simulink model "c00002"  (R2018a)
settings: Solver=FixedStepAuto  StartTime=0.0  StopTime=300  FixedStep=0.1  RelTol=1e-3
undefined symbols (not defined in the file): A1, hmax, R1, R2, TempThreshold
settings Model: Creator=aarrieta  LastModifiedBy=umarkiegi

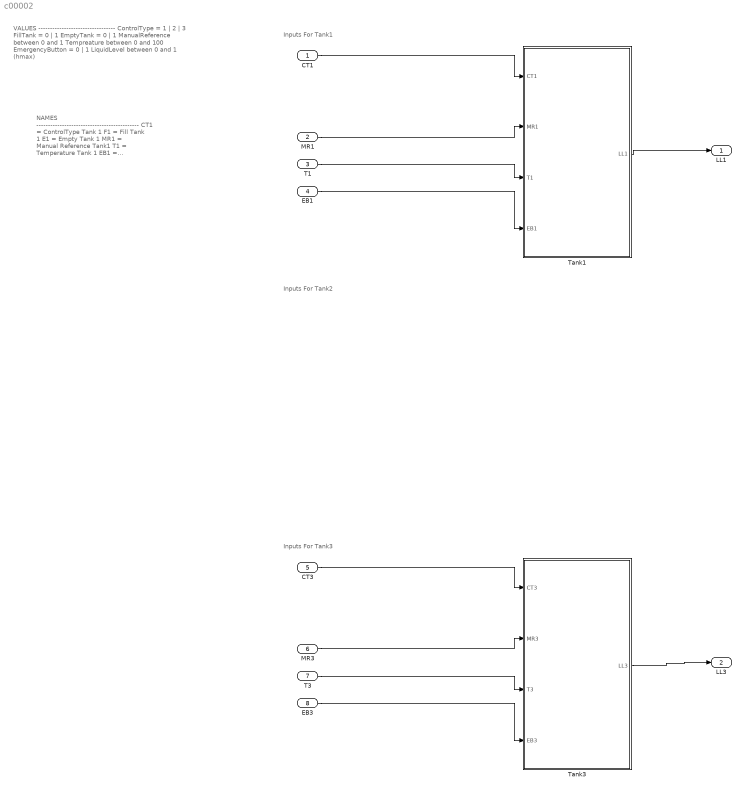
== system c00002 ==
  note: Inputs For Tank1
  note: VALUES
      | ---------------------------------
      | ControlType = 1 | 2 | 3
      | FillTank = 0 | 1
      | EmptyTank = 0 | 1
      | ManualReference between 0 and 1
      | Tempreature between 0 and 100
      | EmergencyButton = 0 | 1
      | LiquidLevel between 0 and 1 (hmax)
  note: NAMES
      | --------------------------------------------
      | CT1 = ControlType Tank 1
      | F1 = Fill Tank 1
      | E1 = Empty Tank 1
      | MR1 = Manual Reference Tank1
      | T1 = Temperature Tank 1
      | EB1 = Emergency Button Tank 1
      | LL1 = Liquid Level 1
  note: Inputs For Tank2
  note: Inputs For Tank3
  CT1 : Inport
  MR1 : Inport  Port=2
  T1 : Inport  Port=3
  EB1 : Inport  Port=4
  CT3 : Inport  Port=5
  MR3 : Inport  Port=6
  T3 : Inport  Port=7
  EB3 : Inport  Port=8
  Tank1 : Subsystem
  Tank3 : Subsystem
  LL1 : Outport
  LL3 : Outport  Port=2
  wires:
  Tank1/1(LL1) -> LL1/1
  CT1/1 -> Tank1/1(CT1)
  MR1/1 -> Tank1/2(MR1)
  T1/1 -> Tank1/3(T1)
  EB1/1 -> Tank1/4(EB1)
  Tank3/1(LL3) -> LL3/1
  MR3/1 -> Tank3/2(MR3)
  T3/1 -> Tank3/3(T3)
  EB3/1 -> Tank3/4(EB3)
  CT3/1 -> Tank3/1(CT3)

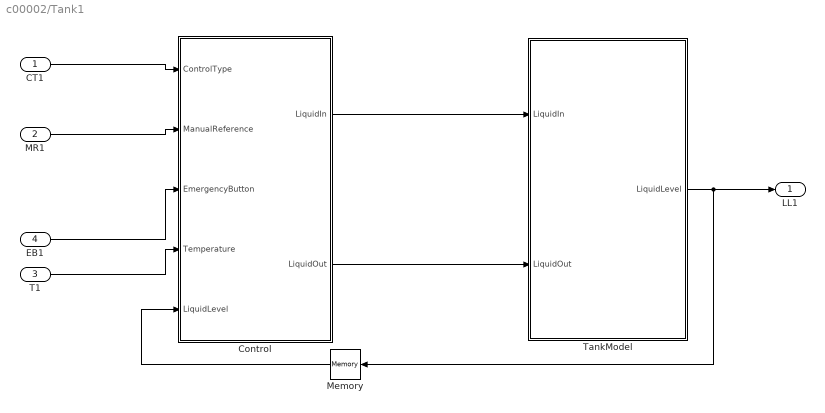
== system c00002/Tank1 ==
  CT1 : Inport
  MR1 : Inport  Port=2
  T1 : Inport  Port=3
  EB1 : Inport  Port=4
  Control : Subsystem
  Memory : Memory
  TankModel : Subsystem
  LL1 : Outport
  wires:
  TankModel/1(LiquidLevel) -> Memory/1, LL1/1
  Control/2(LiquidOut) -> TankModel/2(LiquidOut)
  Memory/1 -> Control/5(LiquidLevel)
  MR1/1 -> Control/2(ManualReference)
  CT1/1 -> Control/1(ControlType)
  EB1/1 -> Control/3(EmergencyButton)
  T1/1 -> Control/4(Temperature)
  Control/1(LiquidIn) -> TankModel/1(LiquidIn)

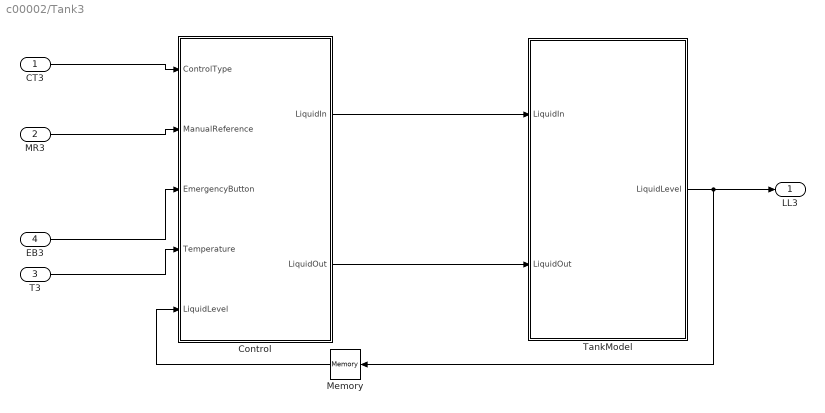
== system c00002/Tank3 ==
  CT3 : Inport
  MR3 : Inport  Port=2
  T3 : Inport  Port=3
  EB3 : Inport  Port=4
  Control : Subsystem
  Memory : Memory
  TankModel : Subsystem
  LL3 : Outport
  wires:
  TankModel/1(LiquidLevel) -> Memory/1, LL3/1
  Control/2(LiquidOut) -> TankModel/2(LiquidOut)
  Memory/1 -> Control/5(LiquidLevel)
  MR3/1 -> Control/2(ManualReference)
  CT3/1 -> Control/1(ControlType)
  EB3/1 -> Control/3(EmergencyButton)
  T3/1 -> Control/4(Temperature)
  Control/1(LiquidIn) -> TankModel/1(LiquidIn)

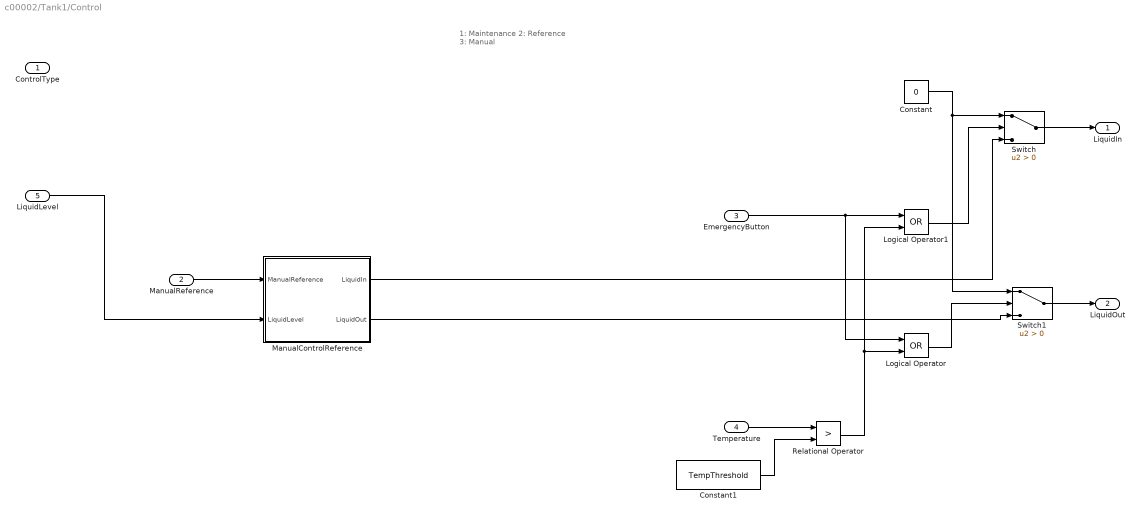
== system c00002/Tank1/Control ==
  note: 1: Maintenance
      | 2: Reference
      | 3: Manual
  ControlType : Inport
  ManualReference : Inport  Port=2
  EmergencyButton : Inport  Port=3
  Temperature : Inport  Port=4
  LiquidLevel : Inport  Port=5
  Constant : Constant  Value=0
  Constant1 : Constant  Value=TempThreshold
  Logical Operator : Logic  Operator=OR  AllPortsSameDT=off  OutDataTypeStr=boolean
  Logical Operator1 : Logic  Operator=OR  AllPortsSameDT=off  OutDataTypeStr=boolean
  ManualControlReference : Subsystem
  Relational Operator : RelationalOperator  Operator=>  OutDataTypeStr=boolean  RndMeth=Simplest
  Switch : Switch  Criteria=u2 > Threshold
  Switch1 : Switch  Criteria=u2 > Threshold
  LiquidIn : Outport
  LiquidOut : Outport  Port=2
  wires:
  ManualReference/1 -> ManualControlReference/1(ManualReference)
  LiquidLevel/1 -> ManualControlReference/2(LiquidLevel)
  Switch/1 -> LiquidIn/1
  Switch1/1 -> LiquidOut/1
  Constant/1 -> Switch1/1, Switch/1
  EmergencyButton/1 -> Logical Operator/1, Logical Operator1/1
  Relational Operator/1 -> Logical Operator1/2, Logical Operator/2
  Logical Operator/1 -> Switch1/2
  Logical Operator1/1 -> Switch/2
  Temperature/1 -> Relational Operator/1
  Constant1/1 -> Relational Operator/2
  ManualControlReference/1(LiquidIn) -> Switch/3
  ManualControlReference/2(LiquidOut) -> Switch1/3

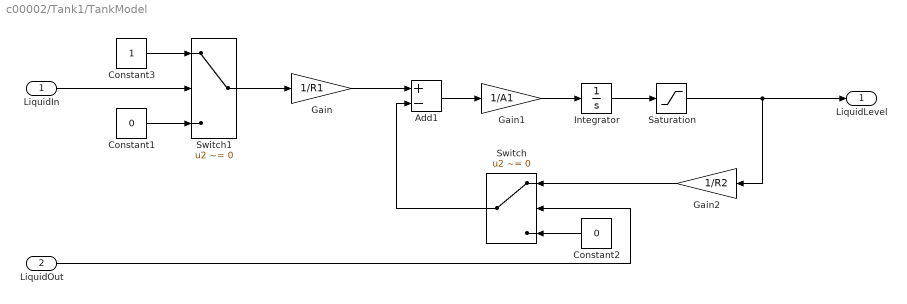
== system c00002/Tank1/TankModel ==
  LiquidIn : Inport
  LiquidOut : Inport  Port=2
  Add1 : Sum  Inputs=+-
  Constant1 : Constant  Value=0
  Constant2 : Constant  Value=0
  Constant3 : Constant
  Gain : Gain  Gain=1/R1
  Gain1 : Gain  Gain=1/A1
  Gain2 : Gain  Gain=1/R2
  Integrator : Integrator
  Saturation : Saturate  UpperLimit=hmax  LowerLimit=0
  Switch : Switch  Criteria=u2 ~= 0
  Switch1 : Switch  Criteria=u2 ~= 0
  LiquidLevel : Outport
  wires:
  Saturation/1 -> LiquidLevel/1, Gain2/1
  LiquidOut/1 -> Switch/2
  Add1/1 -> Gain1/1
  Gain2/1 -> Switch/1
  LiquidIn/1 -> Switch1/2
  Switch/1 -> Add1/2
  Switch1/1 -> Gain/1
  Constant2/1 -> Switch/3
  Constant3/1 -> Switch1/1
  Integrator/1 -> Saturation/1
  Gain1/1 -> Integrator/1
  Gain/1 -> Add1/1
  Constant1/1 -> Switch1/3

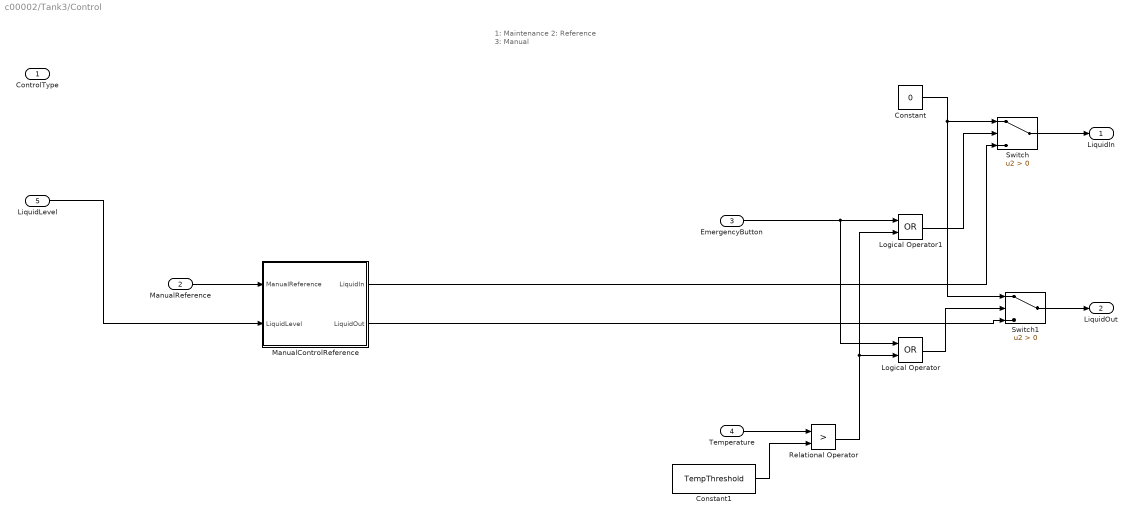
== system c00002/Tank3/Control ==
  note: 1: Maintenance
      | 2: Reference
      | 3: Manual
  ControlType : Inport
  ManualReference : Inport  Port=2
  EmergencyButton : Inport  Port=3
  Temperature : Inport  Port=4
  LiquidLevel : Inport  Port=5
  Constant : Constant  Value=0
  Constant1 : Constant  Value=TempThreshold
  Logical Operator : Logic  Operator=OR  AllPortsSameDT=off  OutDataTypeStr=boolean
  Logical Operator1 : Logic  Operator=OR  AllPortsSameDT=off  OutDataTypeStr=boolean
  ManualControlReference : Subsystem
  Relational Operator : RelationalOperator  Operator=>  OutDataTypeStr=boolean  RndMeth=Simplest
  Switch : Switch  Criteria=u2 > Threshold
  Switch1 : Switch  Criteria=u2 > Threshold
  LiquidIn : Outport
  LiquidOut : Outport  Port=2
  wires:
  ManualReference/1 -> ManualControlReference/1(ManualReference)
  LiquidLevel/1 -> ManualControlReference/2(LiquidLevel)
  Switch/1 -> LiquidIn/1
  Switch1/1 -> LiquidOut/1
  Constant/1 -> Switch1/1, Switch/1
  EmergencyButton/1 -> Logical Operator/1, Logical Operator1/1
  Relational Operator/1 -> Logical Operator1/2, Logical Operator/2
  Logical Operator/1 -> Switch1/2
  Logical Operator1/1 -> Switch/2
  Temperature/1 -> Relational Operator/1
  Constant1/1 -> Relational Operator/2
  ManualControlReference/1(LiquidIn) -> Switch/3
  ManualControlReference/2(LiquidOut) -> Switch1/3

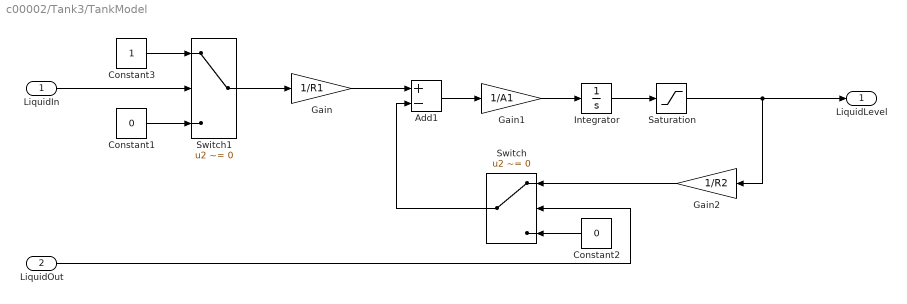
== system c00002/Tank3/TankModel ==
  LiquidIn : Inport
  LiquidOut : Inport  Port=2
  Add1 : Sum  Inputs=+-
  Constant1 : Constant  Value=0
  Constant2 : Constant  Value=0
  Constant3 : Constant
  Gain : Gain  Gain=1/R1
  Gain1 : Gain  Gain=1/A1
  Gain2 : Gain  Gain=1/R2
  Integrator : Integrator
  Saturation : Saturate  UpperLimit=hmax  LowerLimit=0
  Switch : Switch  Criteria=u2 ~= 0
  Switch1 : Switch  Criteria=u2 ~= 0
  LiquidLevel : Outport
  wires:
  Saturation/1 -> LiquidLevel/1, Gain2/1
  LiquidOut/1 -> Switch/2
  Add1/1 -> Gain1/1
  Gain2/1 -> Switch/1
  LiquidIn/1 -> Switch1/2
  Switch/1 -> Add1/2
  Switch1/1 -> Gain/1
  Constant2/1 -> Switch/3
  Constant3/1 -> Switch1/1
  Integrator/1 -> Saturation/1
  Gain1/1 -> Integrator/1
  Gain/1 -> Add1/1
  Constant1/1 -> Switch1/3

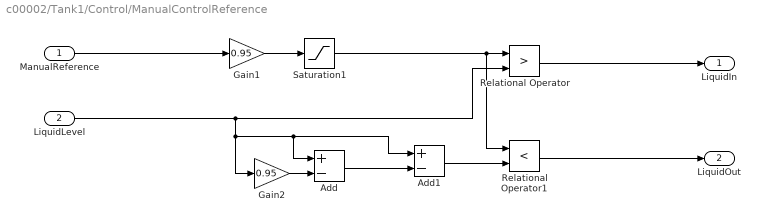
== system c00002/Tank1/Control/ManualControlReference ==
  ManualReference : Inport
  LiquidLevel : Inport  Port=2
  Add : Sum  Inputs=+-
  Add1 : Sum  Inputs=+-
  Gain1 : Gain  Gain=0.95
  Gain2 : Gain  Gain=0.95
  Relational Operator : RelationalOperator  Operator=>  OutDataTypeStr=boolean  RndMeth=Simplest
  Relational Operator1 : RelationalOperator  Operator=<  OutDataTypeStr=boolean  RndMeth=Simplest
  Saturation1 : Saturate  UpperLimit=hmax*0.9  LowerLimit=0
  LiquidIn : Outport
  LiquidOut : Outport  Port=2
  wires:
  LiquidLevel/1 -> Relational Operator/2, Add/1, Add1/1, Gain2/1
  Relational Operator/1 -> LiquidIn/1
  Relational Operator1/1 -> LiquidOut/1
  Add/1 -> Add1/2
  Add1/1 -> Relational Operator1/2
  Gain1/1 -> Saturation1/1
  Gain2/1 -> Add/2
  ManualReference/1 -> Gain1/1
  Saturation1/1 -> Relational Operator1/1, Relational Operator/1

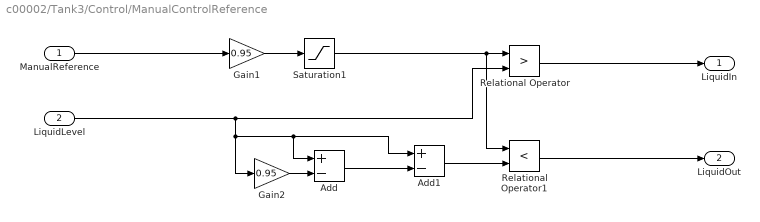
== system c00002/Tank3/Control/ManualControlReference ==
  ManualReference : Inport
  LiquidLevel : Inport  Port=2
  Add : Sum  Inputs=+-
  Add1 : Sum  Inputs=+-
  Gain1 : Gain  Gain=0.95
  Gain2 : Gain  Gain=0.95
  Relational Operator : RelationalOperator  Operator=>  OutDataTypeStr=boolean  RndMeth=Simplest
  Relational Operator1 : RelationalOperator  Operator=<  OutDataTypeStr=boolean  RndMeth=Simplest
  Saturation1 : Saturate  UpperLimit=hmax*0.9  LowerLimit=0
  LiquidIn : Outport
  LiquidOut : Outport  Port=2
  wires:
  LiquidLevel/1 -> Relational Operator/2, Add/1, Add1/1, Gain2/1
  Relational Operator/1 -> LiquidIn/1
  Relational Operator1/1 -> LiquidOut/1
  Add/1 -> Add1/2
  Add1/1 -> Relational Operator1/2
  Gain1/1 -> Saturation1/1
  Gain2/1 -> Add/2
  ManualReference/1 -> Gain1/1
  Saturation1/1 -> Relational Operator1/1, Relational Operator/1
